simulink model "model3"  (R2022a)
settings: Solver=FixedStepAuto  StartTime=0.0  StopTime=100  FixedStep=1  RelTol=1e-3
values from neighbouring files (symbols this model uses):
  testMap = [0  0  0; 0  1  0; 0  0  0]    [aufgabe2.mat]
settings Model: Creator=JadKHaddad  LastModifiedBy=JadKHaddad

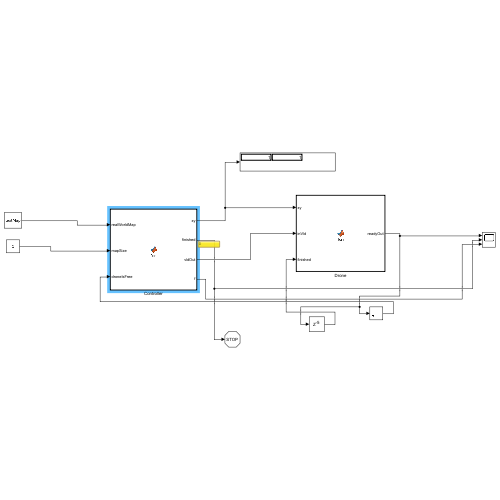
[thumbnail: Simulink's stored preview of the top-level diagram]
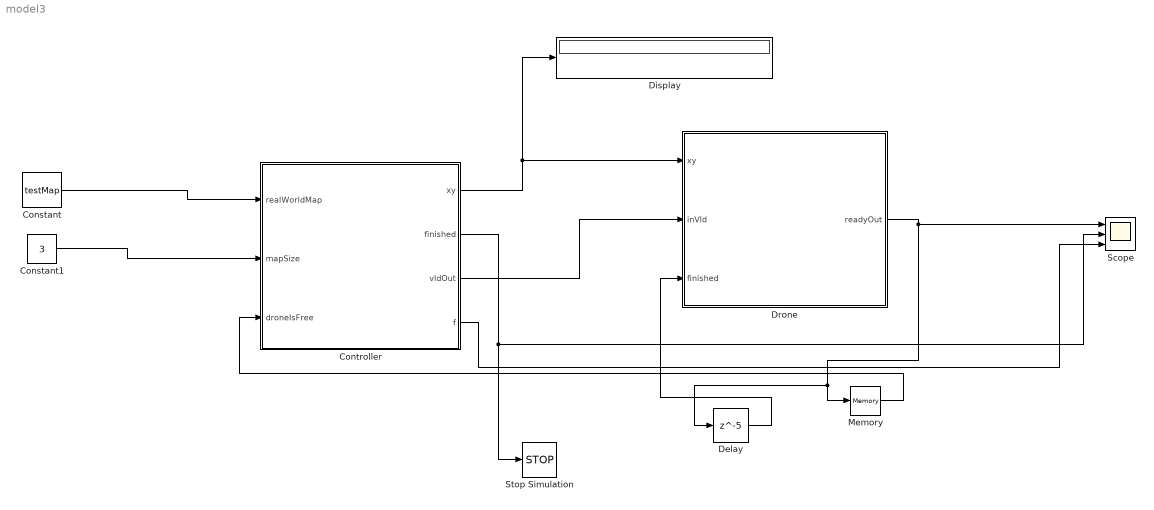
== system model3 ==
  Constant : Constant  Value=testMap  VectorParams1D=off
  Constant1 : Constant  Value=3
  Controller : MATLAB Function  TreatAsAtomicUnit=on
  Delay : Delay  DelayLength=5
  Display : Display
  Drone : MATLAB Function  TreatAsAtomicUnit=on
  Memory : Memory
  Scope : Scope  NumInputPorts=3
  Stop Simulation : Stop
  wires:
  Constant/1 -> Controller/1(realWorldMap)
  Controller/3(vldOut) -> Drone/2(inVld)
  Constant1/1 -> Controller/2(mapSize)
  Controller/1(xy) -> Display/1, Drone/1(xy)
  Controller/2(finished) -> Stop Simulation/1, Scope/2
  Drone/1(readyOut) -> Memory/1, Delay/1, Scope/1
  Memory/1 -> Controller/3(droneIsFree)
  Delay/1 -> Drone/3(finished)
  Controller/4(f) -> Scope/3

== matlab function model3/Drone ==
  data: xy input; readyOut output; inVld input; finished input
function readyOut = fcn(xy, inVld, finished)

persistent ready
if isempty(ready)
    ready = 1;
end

if finished == 1
    ready = 1;
end
if inVld == 1 && ready == 1
    ready = 0;
end

readyOut = ready;

== matlab function model3/Controller ==
  data: realWorldMap input; mapSize input; xy output; droneIsFree input; finished output; vldOut output; f output
function [xy, finished, vldOut, f] = fcn(realWorldMap, mapSize, droneIsFree)
    persistent index
    persistent indexLimit
    persistent path
    persistent lastXY
    


    if isempty(index)
        index = 1;
    end
    if isempty(indexLimit)
        indexLimit = 2;
    end
    if isempty(path)
        path = ones(mapSize*mapSize,2);
    end
    if isempty(lastXY)
        lastXY = [-1 -1];
    end

    
    vldOut = 0;
    finished = 0;
    xy = [1 1];
    f = droneIsFree;

    if index >= mapSize*mapSize
        finished = 1;
        return
    end
    %update path
    x = lastXY(1, 1);
    y = lastXY(1, 2);
    if droneIsFree == 1 && ~isequal(x, -1)
        %update path
        disp("updating path");

        if realWorldMap(x,y) == 0
            if x + 1 <= length(realWorldMap) && realWorldMap(x + 1, y) == 0 && containsFunc(path, x + 1, y) == 0
                newRow = [x+1 y];
                path(indexLimit,:) = newRow;
                indexLimit = indexLimit + 1;
            end
            
            if y + 1 <= length(realWorldMap) && realWorldMap(x, y + 1) == 0 && containsFunc(path, x, y + 1) == 0
                newRow = [x y+1];
                path(indexLimit,:) = newRow;
                indexLimit = indexLimit + 1;
            end
            
            if x - 1 >= 1 && realWorldMap(x - 1, y) == 0 && containsFunc(path, x - 1, y) == 0
                newRow = [x-1 y];
                path(indexLimit-1,:) = newRow;
                indexLimit = indexLimit + 1;
            end
            
            if y - 1 >= 1 && realWorldMap(x, y-1) == 0 && containsFunc(path, x, y - 1) == 0
                newRow = [x y-1];
                path(indexLimit,:) = newRow;
                indexLimit = indexLimit + 1;
            end
        end
        disp(path);
        disp(indexLimit);
    end

    if index < indexLimit
        if droneIsFree == 1
            vldOut = 1;
            %get next pos
            xy = path(index,:);
            lastXY = xy;
            index = index + 1;
            
        end
    else
        if droneIsFree == 1
            finished = 1;
        end
    end
